simulink model "fullstate_sim"  (R2020a)
settings: Solver=FixedStepAuto  StartTime=0.0  StopTime=5  FixedStep=0.002  RelTol=1e-6
undefined symbols (not defined in the file): icd, K, sysd_full
settings Model: Creator=Jasper  LastModifiedBy=Jasper

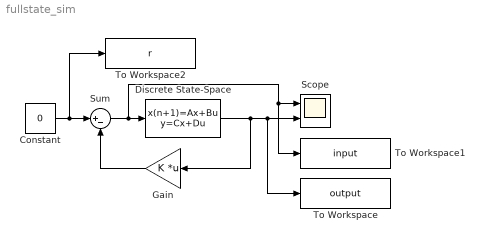
== system fullstate_sim ==
  Constant : Constant  Value=0
  Discrete State-Space : DiscreteStateSpace  A=sysd_full.A  B=sysd_full.B  C=sysd_full.C  D=sysd_full.D  InitialCondition=icd  SampleTime=-1
  Gain : Gain  Gain=K  Multiplication=Matrix(K*u)
  Scope : Scope  NumInputPorts=2
  Sum : Sum  Inputs=|+-
  To Workspace : ToWorkspace  VariableName=output  SaveFormat=Timeseries  SampleTime=-1
  To Workspace1 : ToWorkspace  VariableName=input  SaveFormat=Timeseries  SampleTime=-1
  To Workspace2 : ToWorkspace  VariableName=r  SaveFormat=Timeseries  SampleTime=-1
  wires:
  Discrete State-Space/1 -> To Workspace/1, Scope/2, Gain/1
  Gain/1 -> Sum/2
  Sum/1 -> Discrete State-Space/1, To Workspace1/1, Scope/1
  Constant/1 -> To Workspace2/1, Sum/1
